simulink model "c00001M_harness"  (R2018a)
settings: Solver=ode3  StartTime=0.0  StopTime=10.0  RelTol=1e-3  EnableMultiTasking=on
undefined symbols (not defined in the file): b, DiscIntNeverNeededParam, J, K, L, R, sigbuilder_block
settings Model: Creator=aarrieta  LastModifiedBy=umarkiegi
settings DataIOCC: LimitDataPoints=on  SaveFormat=Array
settings OptimizationCC: LifeSpan=inf
settings DebuggingCC: UnderspecifiedInitializationDetection=Classic  MergeDetectMultiDrivingBlocksExec=none  SolverPrmCheckMsg=warning  StateNameClashWarn=warning  SFUnexpectedBacktrackingDiag=warning  SFNoUnconditionalDefaultTransitionDiag=warning  SFExecutionAtInitializationDiag=none
settings HardwareCC: ProdBitPerPointer=32  ProdBitPerSizeT=32  ProdBitPerPtrDiffT=32  ProdLargestAtomicFloat=None  ProdIntDivRoundTo=Undefined  ProdEndianess=Unspecified  ProdWordSize=32  ProdHWDeviceType=32-bit Generic
settings ModelReferenceCC: PropagateSignalLabelsOutOfModel=off
settings CodeAppCC: StateflowObjectComments=on
settings GRTTargetCC: TargetLangStandard=C89/C90 (ANSI)  GeneratePreprocessorConditionals=Disable all
settings ConfigComp: CovMetricSettings=dw  CovHtmlReporting=on  CovSaveCumulativeToWorkspaceVar=on  CovSaveSingleToWorkspaceVar=on  CovExternalEMLEnable=off  DVMaxTestCaseSteps=20  DVTestSuiteOptimization=CombinedObjectives (Nonlinear Extended)  DVDetectFloatOverflow=off

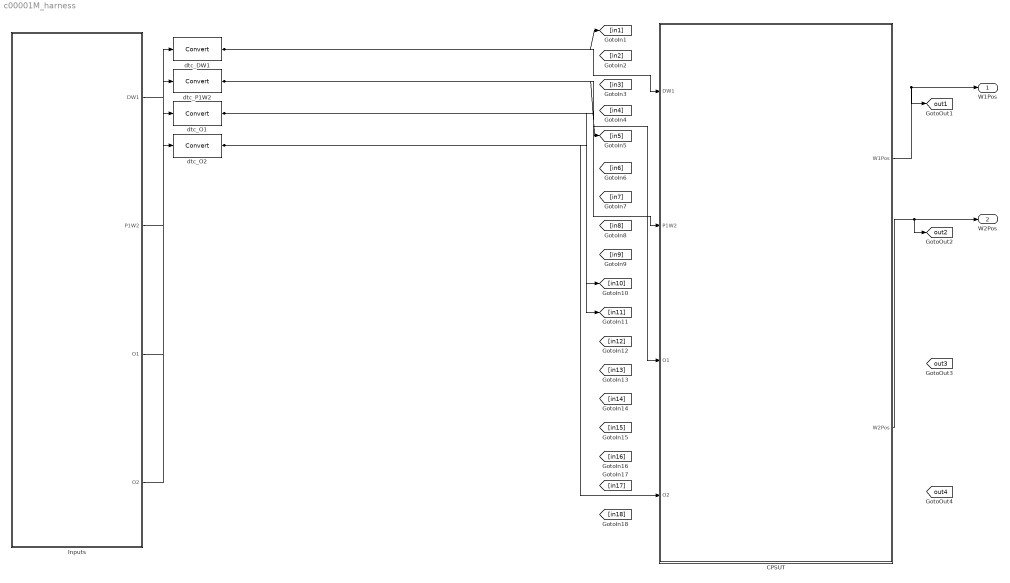
== system c00001M_harness ==
  CPSUT : Subsystem
  Inputs : Subsystem  Tag=STV Subsys  LoadFcn=sigbuilder_block('load');  StartFcn=sigbuilder_block('start');  StopFcn=sigbuilder_block('stop');  ClipboardFcn=sigbuilder_block('clipboard');  mask(Sigbuilder block){tuvar=[0:10]}
      mask init:
      | if ~strcmp(get_param(bdroot(gcb),'SimulationStatus'),'stopped'),tuvar = sigbuilder_block('maskInit'); end
      settings: CopyFcn=sigbuilder_block('copy');  DeleteFcn=sigbuilder_block('delete');  ModelCloseFcn=sigbuilder_block('modelClose');  PreSaveFcn=sigbuilder_block('preSave');  PauseFcn=sigbuilder_block('pause');  ContinueFcn=sigbuilder_block('continue');  NameChangeFcn=sigbuilder_block('namechange');  OpenFcn=sigbuilder_block('open');  CloseFcn=sigbuilder_block('close');
      mask Display: plot(0, 0, 100, 100,[2, 2, 32, 32, 2], [68, 8, 8, 68, 68],[32, 2], [38, 38], [32, 19, 2],[53, 60, 44], [32, 17, 17, 2],[16, 16, 31, 31]);txt = getActiveGroup(gcbh);text(2, 100, txt,'verticalAlignment', 'top');
  dtc_DW1 : DataTypeConversion
  dtc_O1 : DataTypeConversion
  dtc_O2 : DataTypeConversion
  dtc_P1W2 : DataTypeConversion
  W1Pos : Outport
  W2Pos : Outport  Port=2
  tag scope: out1=global, out2=global, out3=global, out4=global
  wires:
  CPSUT/2(W2Pos) -> [out2], W2Pos/1
  CPSUT/1(W1Pos) -> [out1], W1Pos/1
  Inputs/1(DW1) -> dtc_DW1/1
  dtc_DW1/1 -> CPSUT/1(DW1), [in1]
  Inputs/2(P1W2) -> dtc_P1W2/1
  dtc_P1W2/1 -> CPSUT/2(P1W2), [in5]
  Inputs/3(O1) -> dtc_O1/1
  dtc_O1/1 -> CPSUT/3(O1), [in10]
  Inputs/4(O2) -> dtc_O2/1
  dtc_O2/1 -> CPSUT/4(O2), [in11]

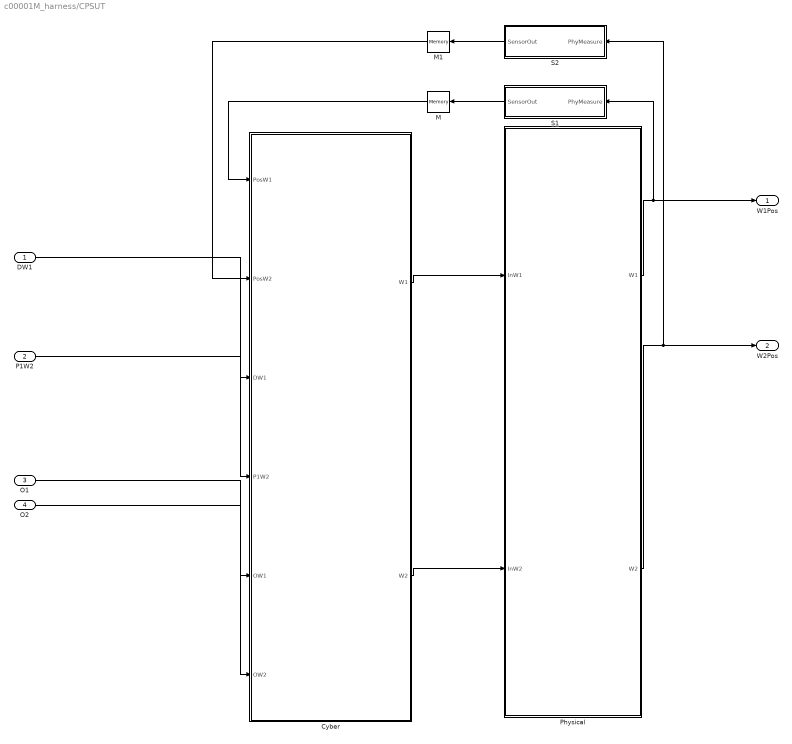
== system c00001M_harness/CPSUT ==
  DW1 : Inport  OutMin=0  OutMax=4  OutDataTypeStr=int8
  P1W2 : Inport  Port=2  OutMin=0  OutMax=4  OutDataTypeStr=int8
  O1 : Inport  Port=3  OutDataTypeStr=boolean
  O2 : Inport  Port=4  OutDataTypeStr=boolean
  Cyber : Subsystem
  M : Memory
  M1 : Memory
  Physical : Subsystem
  S1 : Subsystem
  S2 : Subsystem
  W1Pos : Outport
  W2Pos : Outport  Port=2
  wires:
  S1/1(SensorOut) -> M/1
  Physical/1(W1) -> W1Pos/1, S1/1(PhyMeasure)
  O2/1 -> Cyber/6(OW2)
  O1/1 -> Cyber/5(OW1)
  Cyber/1(W1) -> Physical/1(InW1)
  Cyber/2(W2) -> Physical/2(InW2)
  P1W2/1 -> Cyber/4(P1W2)
  M1/1 -> Cyber/2(PosW2)
  M/1 -> Cyber/1(PosW1)
  DW1/1 -> Cyber/3(DW1)
  Physical/2(W2) -> W2Pos/1, S2/1(PhyMeasure)
  S2/1(SensorOut) -> M1/1

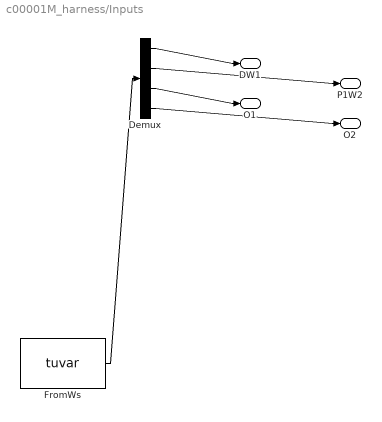
== system c00001M_harness/Inputs ==
  Demux : Demux  Tag=STV Demux
  FromWs : FromWorkspace  Tag=STV FromWs  VariableName=tuvar  SampleTime=0
      SigBuilderData=|
      | dataSet(1).timeRange = [0 20]
      | dataSet(1).name = 'Test Case 1'
      | dataSet(2).timeRange = [0 10]
      | dataSet(2).name = 'Test Case 2'
      | dataSet(3).timeRange = [0 8]
      | dataSet(3).name = 'Test Case 3'
      | dataSet(4).timeRange = [0 6]
      | dataSet(4).name = 'Test Case 4'
      | dataSet(5).timeRange = [0 6]
      | dataSet(5).name = 'Test Case 5'
      | dataSet(6).timeRange = [0 6]
      | dataSet(6).name = 'Test Case 6'
      | dataSet(7).timeRange = [0 8]
      | dataSet(7).name = 'Test Case 7'
      | dataSet(8).timeRange = [0 6]
      | dataSet(8).name = 'Test Case 8'
      | dataSet(9).timeRange = [0 6]
      | dataSet(9).name = 'Test Case 9'
      | dataSet(10).timeRange = [0 7]
      | dataSet(10).name = 'Test Case 10'
      | dataSet(11).timeRange = [0 9]
      | dataSet(11).name = 'Test Case 11'
      | dataSet(12).timeRange = [0 8]
      | dataSet(12).name = 'Test Case 12'
      | dataSet(13).timeRange = [0 12]
      | dataSet(13).name = 'Test Case 13'
      | dataSet(14).timeRange = [0 8]
      | dataSet(14).name = 'Test Case 14'
      | dataSet(15).timeRange = [0 8]
      | dataSet(15).name = 'Test Case 15'
      | dataSet(16).timeRange = [0 8]
      | dataSet(16).name = 'Test Case 16'
      | dataSet(17).timeRange = [0 8]
      | dataSet(17).name = 'Test Case 17'
      | dataSet(18).timeRange = [0 8]
      | dataSet(18).name = 'Test Case 18'
      | dataSet(19).timeRange = [0 8]
      | dataSet(19).name = 'Test Case 19'
      | dataSet(20).timeRange = [0 7]
      | dataSet(20).name = 'Test Case 20'
      | dataSet(21).timeRange = [0 7]
      | dataSet(21).name = 'Test Case 21'
      | dataSet(22).timeRange = [0 7]
      | dataSet(22).name = 'Test Case 22'
      | dataSet(23).timeRange = [0 8]
      | dataSet(23).name = 'Test Case 23'
      | dataSet(24).timeRange = [0 8]
      | dataSet(24).name = 'Test Case 24'
      | dataSet(25).timeRange = [0 8]
      | dataSet(25).name = 'Test Case 25'
      | dataSet(26).timeRange = [0 8]
      | dataSet(26).name = 'Test Case 26'
      | sbobj.Name = 'Signal Builder'
      | sbobj.Groups(1).Name = 'Test Case 1'
      | sbobj.Groups(1).Signals(1).Name = 'DW1'
      | sbobj.Groups(1).Signals(1).XData = [0 2 8 11 11 13 16 17 17 19 19 20]
      | sbobj.Groups(1).Signals(1).YData = [1 1 1 1 0 0 0 0 4 4 3 3]
      | sbobj.Groups(1).Signals(2).Name = 'P1W2'
      | sbobj.Groups(1).Signals(2).XData = [0 2 2 8 8 11 11 13 13 16 16 17 17 19 19 20]
      | sbobj.Groups(1).Signals(2).YData = [2 2 2 2 4 4 3 3 1 1 0 0 0 0 0 0]
      | sbobj.Groups(1).Signals(3).Name = 'O1'
      | sbobj.Groups(1).Signals(3).XData = [0 2 2 8 8 11 11 13 13 16 16 17 17 19 19 20]
      | sbobj.Groups(1).Signals(3).YData = [1 1 1 1 1 1 1 1 1 1 0 0 0 0 0 0]
      | sbobj.Groups(1).Signals(4).Name = 'O2'
      | sbobj.Groups(1).Signals(4).XData = [0 2 2 8 8 11 11 13 13 16 16 17 17 19 19 20]
      | sbobj.Groups(1).Signals(4).YData = [0 0 1 1 0 0 0 0 0 0 0 0 0 0 0 0]
      | sbobj.Groups(1).TimeRange = [0 20]
      | sbobj.Groups(2).Name = 'Test Case 2'
      | sbobj.Groups(2).Signals(1).Name = 'DW1'
      | sbobj.Groups(2).Signals(1).XData = [0 3 3 5 5 9 9 10]
      | sbobj.Groups(2).Signals(1).YData = [3 3 3 3 2 2 2 2]
      | sbobj.Groups(2).Signals(2).Name = 'P1W2'
      | sbobj.Groups(2).Signals(2).XData = [0 3 3 5 5 9 9 10]
      | sbobj.Groups(2).Signals(2).YData = [3 3 0 0 0 0 1 1]
      | sbobj.Groups(2).Signals(3).Name = 'O1'
      | sbobj.Groups(2).Signals(3).XData = [0 3 3 5 5 9 9 10]
      | sbobj.Groups(2).Signals(3).YData = [1 1 1 1 0 0 0 0]
      | sbobj.Groups(2).Signals(4).Name = 'O2'
      | sbobj.Groups(2).Signals(4).XData = [0 3 3 5 5 9 9 10]
      | sbobj.Groups(2).Signals(4).YData = [0 0 0 0 0 0 0 0]
      | sbobj.Groups(3).Name = 'Test Case 3'
      | sbobj.Groups(3).Signals(1).Name = 'DW1'
      | sbobj.Groups(3).Signals(1).XData = [0 3 3 4 4 7 7 8]
      | sbobj.Groups(3).Signals(1).YData = [4 4 0 0 1 1 1 1]
      | sbobj.Groups(3).Signals(2).Name = 'P1W2'
      | sbobj.Groups(3).Signals(2).XData = [0 3 3 4 4 7 7 8]
      | sbobj.Groups(3).Signals(2).YData = [4 4 1 1 0 0 3 3]
      | sbobj.Groups(3).Signals(3).Name = 'O1'
      | sbobj.Groups(3).Signals(3).XData = [0 3 3 4 4 7 7 8]
      | sbobj.Groups(3).Signals(3).YData = [0 0 0 0 0 0 0 0]
      | sbobj.Groups(3).Signals(4).Name = 'O2'
      | sbobj.Groups(3).Signals(4).XData = [0 3 3 4 4 7 7 8]
      | sbobj.Groups(3).Signals(4).YData = [0 0 0 0 0 0 0 0]
      | sbobj.Groups(3).TimeRange = [0 8]
      | sbobj.Groups(4).Name = 'Test Case 4'
      | sbobj.Groups(4).Signals(1).Name = 'DW1'
      | sbobj.Groups(4).Signals(1).XData = [0 3 3 5 5 6]
      | sbobj.Groups(4).Signals(1).YData = [4 4 2 2 2 2]
      | sbobj.Groups(4).Signals(2).Name = 'P1W2'
      | sbobj.Groups(4).Signals(2).XData = [0 3 3 5 5 6]
      | sbobj.Groups(4).Signals(2).YData = [1 1 0 0 0 0]
      | sbobj.Groups(4).Signals(3).Name = 'O1'
      | sbobj.Groups(4).Signals(3).XData = [0 3 3 5 5 6]
      | sbobj.Groups(4).Signals(3).YData = [0 0 0 0 0 0]
      | sbobj.Groups(4).Signals(4).Name = 'O2'
      | sbobj.Groups(4).Signals(4).XData = [0 3 3 5 5 6]
      | sbobj.Groups(4).Signals(4).YData = [0 0 0 0 1 1]
      | sbobj.Groups(4).TimeRange = [0 6]
      | sbobj.Groups(5).Name = 'Test Case 5'
      | sbobj.Groups(5).Signals(1).Name = 'DW1'
      | sbobj.Groups(5).Signals(1).XData = [0 3 3 5 5 6]
      | sbobj.Groups(5).Signals(1).YData = [3 3 0 0 3 3]
      | sbobj.Groups(5).Signals(2).Name = 'P1W2'
      | sbobj.Groups(5).Signals(2).XData = [0 3 3 5 5 6]
      | sbobj.Groups(5).Signals(2).YData = [4 4 0 0 3 3]
      | sbobj.Groups(5).Signals(3).Name = 'O1'
      | sbobj.Groups(5).Signals(3).XData = [0 3 3 5 5 6]
      | sbobj.Groups(5).Signals(3).YData = [0 0 0 0 1 1]
      | sbobj.Groups(5).Signals(4).Name = 'O2'
      | sbobj.Groups(5).Signals(4).XData = [0 3 3 5 5 6]
      | sbobj.Groups(5).Signals(4).YData = [1 1 0 0 0 0]
      | sbobj.Groups(5).TimeRange = [0 6]
      | sbobj.Groups(6).Name = 'Test Case 6'
      | sbobj.Groups(6).Signals(1).Name = 'DW1'
      | sbobj.Groups(6).Signals(1).XData = [0 3 3 5 5 6]
      | sbobj.Groups(6).Signals(1).YData = [1 1 1 1 0 0]
      | sbobj.Groups(6).Signals(2).Name = 'P1W2'
      | sbobj.Groups(6).Signals(2).XData = [0 3 3 5 5 6]
      | sbobj.Groups(6).Signals(2).YData = [4 4 2 2 0 0]
      | sbobj.Groups(6).Signals(3).Name = 'O1'
      | sbobj.Groups(6).Signals(3).XData = [0 3 3 5 5 6]
      | sbobj.Groups(6).Signals(3).YData = [1 1 1 1 1 1]
      | sbobj.Groups(6).Signals(4).Name = 'O2'
      | sbobj.Groups(6).Signals(4).XData = [0 3 3 5 5 6]
      | sbobj.Groups(6).Signals(4).YData = [0 0 0 0 1 1]
      | sbobj.Groups(6).TimeRange = [0 6]
      | sbobj.Groups(7).Name = 'Test Case 7'
      | sbobj.Groups(7).Signals(1).Name = 'DW1'
      | sbobj.Groups(7).Signals(1).XData = [0 3 3 4 4 7 7 8]
      | sbobj.Groups(7).Signals(1).YData = [1 1 1 1 1 1 3 3]
      | sbobj.Groups(7).Signals(2).Name = 'P1W2'
      | sbobj.Groups(7).Signals(2).XData = [0 3 3 4 4 7 7 8]
      | sbobj.Groups(7).Signals(2).YData = [4 4 3 3 2 2 0 0]
      | sbobj.Groups(7).Signals(3).Name = 'O1'
      | sbobj.Groups(7).Signals(3).XData = [0 3 3 4 4 7 7 8]
      | sbobj.Groups(7).Signals(3).YData = [1 1 1 1 1 1 0 0]
      | sbobj.Groups(7).Signals(4).Name = 'O2'
      | sbobj.Groups(7).Signals(4).XData = [0 3 3 4 4 7 7 8]
      | sbobj.Groups(7).Signals(4).YData = [0 0 0 0 0 0 1 1]
      | sbobj.Groups(7).TimeRange = [0 8]
      | sbobj.Groups(8).Name = 'Test Case 8'
      | sbobj.Groups(8).Signals(1).Name = 'DW1'
      | sbobj.Groups(8).Signals(1).XData = [0 2 2 3 3 5 5 6]
      | sbobj.Groups(8).Signals(1).YData = [1 1 2 2 2 2 2 2]
      | sbobj.Groups(8).Signals(2).Name = 'P1W2'
      | sbobj.Groups(8).Signals(2).XData = [0 2 2 3 3 5 5 6]
      | sbobj.Groups(8).Signals(2).YData = [4 4 3 3 1 1 3 3]
      | sbobj.Groups(8).Signals(3).Name = 'O1'
      | sbobj.Groups(8).Signals(3).XData = [0 2 2 3 3 5 5 6]
      | sbobj.Groups(8).Signals(3).YData = [1 1 1 1 1 1 0 0]
      | sbobj.Groups(8).Signals(4).Name = 'O2'
      | sbobj.Groups(8).Signals(4).XData = [0 2 2 3 3 5 5 6]
      | sbobj.Groups(8).Signals(4).YData = [0 0 1 1 0 0 0 0]
      | sbobj.Groups(8).TimeRange = [0 6]
      | sbobj.Groups(9).Name = 'Test Case 9'
      | sbobj.Groups(9).Signals(1).Name = 'DW1'
      | sbobj.Groups(9).Signals(1).XData = [0 2 2 3 3 5 5 6]
      | sbobj.Groups(9).Signals(1).YData = [1 1 4 4 3 3 2 2]
      | sbobj.Groups(9).Signals(2).Name = 'P1W2'
      | sbobj.Groups(9).Signals(2).XData = [0 2 2 3 3 5 5 6]
      | sbobj.Groups(9).Signals(2).YData = [4 4 0 0 0 0 1 1]
      | sbobj.Groups(9).Signals(3).Name = 'O1'
      | sbobj.Groups(9).Signals(3).XData = [0 2 2 3 3 5 5 6]
      | sbobj.Groups(9).Signals(3).YData = [1 1 1 1 0 0 1 1]
      | sbobj.Groups(9).Signals(4).Name = 'O2'
      | sbobj.Groups(9).Signals(4).XData = [0 2 2 3 3 5 5 6]
      | sbobj.Groups(9).Signals(4).YData = [0 0 1 1 0 0 1 1]
      | sbobj.Groups(9).TimeRange = [0 6]
      | sbobj.Groups(10).Name = 'Test Case 10'
      | sbobj.Groups(10).Signals(1).Name = 'DW1'
      | sbobj.Groups(10).Signals(1).XData = [0 2 2 3 3 6 6 7]
      | sbobj.Groups(10).Signals(1).YData = [1 1 3 3 2 2 0 0]
      | sbobj.Groups(10).Signals(2).Name = 'P1W2'
      | sbobj.Groups(10).Signals(2).XData = [0 2 2 3 3 6 6 7]
      | sbobj.Groups(10).Signals(2).YData = [4 4 0 0 0 0 1 1]
      | sbobj.Groups(10).Signals(3).Name = 'O1'
      | sbobj.Groups(10).Signals(3).XData = [0 2 2 3 3 6 6 7]
      | sbobj.Groups(10).Signals(3).YData = [1 1 1 1 0 0 0 0]
      | sbobj.Groups(10).Signals(4).Name = 'O2'
      | sbobj.Groups(10).Signals(4).XData = [0 2 2 3 3 6 6 7]
      | sbobj.Groups(10).Signals(4).YData = [0 0 1 1 0 0 0 0]
      | sbobj.Groups(10).TimeRange = [0 7]
      | sbobj.Groups(11).Name = 'Test Case 11'
      | sbobj.Groups(11).Signals(1).Name = 'DW1'
      | sbobj.Groups(11).Signals(1).XData = [0 4 4 5 5 7 7 8 8 9]
      | sbobj.Groups(11).Signals(1).YData = [3 3 1 1 0 0 2 2 3 3]
      | sbobj.Groups(11).Signals(2).Name = 'P1W2'
      | sbobj.Groups(11).Signals(2).XData = [0 4 4 5 5 7 7 8 8 9]
      | sbobj.Groups(11).Signals(2).YData = [4 4 0 0 0 0 2 2 3 3]
      | sbobj.Groups(11).Signals(3).Name = 'O1'
      | sbobj.Groups(11).Signals(3).XData = [0 4 4 5 5 7 7 8 8 9]
      | sbobj.Groups(11).Signals(3).YData = [0 0 0 0 0 0 0 0 1 1]
      | sbobj.Groups(11).Signals(4).Name = 'O2'
      | sbobj.Groups(11).Signals(4).XData = [0 4 4 5 5 7 7 8 8 9]
      | sbobj.Groups(11).Signals(4).YData = [1 1 0 0 0 0 0 0 1 1]
      | sbobj.Groups(11).TimeRange = [0 9]
      | sbobj.Groups(12).Name = 'Test Case 12'
      | sbobj.Groups(12).Signals(1).Name = 'DW1'
      | sbobj.Groups(12).Signals(1).XData = [0 4 4 6 6 7 7 8]
      | sbobj.Groups(12).Signals(1).YData = [3 3 4 4 1 1 3 3]
      | sbobj.Groups(12).Signals(2).Name = 'P1W2'
      | sbobj.Groups(12).Signals(2).XData = [0 4 4 6 6 7 7 8]
      | sbobj.Groups(12).Signals(2).YData = [4 4 0 0 1 1 2 2]
      | sbobj.Groups(12).Signals(3).Name = 'O1'
      | sbobj.Groups(12).Signals(3).XData = [0 4 4 6 6 7 7 8]
      | sbobj.Groups(12).Signals(3).YData = [0 0 0 0 1 1 0 0]
      | sbobj.Groups(12).Signals(4).Name = 'O2'
      | sbobj.Groups(12).Signals(4).XData = [0 4 4 6 6 7 7 8]
      | sbobj.Groups(12).Signals(4).YData = [1 1 0 0 0 0 1 1]
      | sbobj.Groups(12).TimeRange = [0 8]
      | sbobj.Groups(13).Name = 'Test Case 13'
      | sbobj.Groups(13).Signals(1).Name = 'DW1'
      | sbobj.Groups(13).Signals(1).XData = [0 2 2 3 3 5 5 6 6 8 8 11 11 12]
      | sbobj.Groups(13).Signals(1).YData = [4 4 4 4 0 0 1 1 1 1 4 4 2 2]
      | sbobj.Groups(13).Signals(2).Name = 'P1W2'
      | sbobj.Groups(13).Signals(2).XData = [0 2 2 3 3 5 5 6 6 8 8 11 11 12]
      | sbobj.Groups(13).Signals(2).YData = [1 1 3 3 4 4 2 2 3 3 0 0 1 1]
      | sbobj.Groups(13).Signals(3).Name = 'O1'
      | sbobj.Groups(13).Signals(3).XData = [0 2 2 3 3 5 5 6 6 8 8 11 11 12]
      | sbobj.Groups(13).Signals(3).YData = [0 0 1 1 1 1 1 1 1 1 1 1 0 0]
      | sbobj.Groups(13).Signals(4).Name = 'O2'
      | sbobj.Groups(13).Signals(4).XData = [0 2 2 3 3 5 5 6 6 8 8 11 11 12]
      | sbobj.Groups(13).Signals(4).YData = [0 0 1 1 0 0 0 0 0 0 0 0 1 1]
      | sbobj.Groups(13).TimeRange = [0 12]
      | sbobj.Groups(14).Name = 'Test Case 14'
      | sbobj.Groups(14).Signals(1).Name = 'DW1'
      | sbobj.Groups(14).Signals(1).XData = [0 3 3 4 4 5 5 7 7 8]
      | sbobj.Groups(14).Signals(1).YData = [4 4 0 0 1 1 4 4 3 3]
      | sbobj.Groups(14).Signals(2).Name = 'P1W2'
      | sbobj.Groups(14).Signals(2).XData = [0 3 3 4 4 5 5 7 7 8]
      | sbobj.Groups(14).Signals(2).YData = [4 4 1 1 0 0 0 0 2 2]
      | sbobj.Groups(14).Signals(3).Name = 'O1'
      | sbobj.Groups(14).Signals(3).XData = [0 3 3 4 4 5 5 7 7 8]
      | sbobj.Groups(14).Signals(3).YData = [0 0 0 0 0 0 0 0 0 0]
      | sbobj.Groups(14).Signals(4).Name = 'O2'
      | sbobj.Groups(14).Signals(4).XData = [0 3 3 4 4 5 5 7 7 8]
      | sbobj.Groups(14).Signals(4).YData = [0 0 0 0 0 0 0 0 1 1]
      | sbobj.Groups(14).TimeRange = [0 8]
      | sbobj.Groups(15).Name = 'Test Case 15'
      | sbobj.Groups(15).Signals(1).Name = 'DW1'
      | sbobj.Groups(15).Signals(1).XData = [0 3 3 4 4 5 5 7 7 8]
      | sbobj.Groups(15).Signals(1).YData = [4 4 0 0 1 1 3 3 0 0]
      | sbobj.Groups(15).Signals(2).Name = 'P1W2'
      | sbobj.Groups(15).Signals(2).XData = [0 3 3 4 4 5 5 7 7 8]
      | sbobj.Groups(15).Signals(2).YData = [4 4 1 1 0 0 0 0 0 0]
      | sbobj.Groups(15).Signals(3).Name = 'O1'
      | sbobj.Groups(15).Signals(3).XData = [0 3 3 4 4 5 5 7 7 8]
      | sbobj.Groups(15).Signals(3).YData = [0 0 0 0 0 0 0 0 1 1]
      | sbobj.Groups(15).Signals(4).Name = 'O2'
      | sbobj.Groups(15).Signals(4).XData = [0 3 3 4 4 5 5 7 7 8]
      | sbobj.Groups(15).Signals(4).YData = [0 0 0 0 0 0 0 0 1 1]
      | sbobj.Groups(15).TimeRange = [0 8]
      | sbobj.Groups(16).Name = 'Test Case 16'
      | sbobj.Groups(16).Signals(1).Name = 'DW1'
      | sbobj.Groups(16).Signals(1).XData = [0 3 3 4 4 5 5 7 7 8]
      | sbobj.Groups(16).Signals(1).YData = [4 4 0 0 1 1 2 2 3 3]
      | sbobj.Groups(16).Signals(2).Name = 'P1W2'
      | sbobj.Groups(16).Signals(2).XData = [0 3 3 4 4 5 5 7 7 8]
      | sbobj.Groups(16).Signals(2).YData = [4 4 1 1 0 0 0 0 4 4]
      | sbobj.Groups(16).Signals(3).Name = 'O1'
      | sbobj.Groups(16).Signals(3).XData = [0 3 3 4 4 5 5 7 7 8]
      | sbobj.Groups(16).Signals(3).YData = [0 0 0 0 0 0 0 0 0 0]
      | sbobj.Groups(16).Signals(4).Name = 'O2'
      | sbobj.Groups(16).Signals(4).XData = [0 3 3 4 4 5 5 7 7 8]
      | sbobj.Groups(16).Signals(4).YData = [0 0 0 0 0 0 0 0 1 1]
      | sbobj.Groups(16).TimeRange = [0 8]
      | sbobj.Groups(17).Name = 'Test Case 17'
      | sbobj.Groups(17).Signals(1).Name = 'DW1'
      | sbobj.Groups(17).Signals(1).XData = [0 4 4 5 5 7 7 8]
      | sbobj.Groups(17).Signals(1).YData = [3 3 4 4 4 4 0 0]
      | sbobj.Groups(17).Signals(2).Name = 'P1W2'
      | sbobj.Groups(17).Signals(2).XData = [0 4 4 5 5 7 7 8]
      | sbobj.Groups(17).Signals(2).YData = [3 3 2 2 4 4 3 3]
      | sbobj.Groups(17).Signals(3).Name = 'O1'
      | sbobj.Groups(17).Signals(3).XData = [0 4 4 5 5 7 7 8]
      | sbobj.Groups(17).Signals(3).YData = [1 1 1 1 1 1 0 0]
      | sbobj.Groups(17).Signals(4).Name = 'O2'
      | sbobj.Groups(17).Signals(4).XData = [0 4 4 5 5 7 7 8]
      | sbobj.Groups(17).Signals(4).YData = [0 0 0 0 0 0 1 1]
      | sbobj.Groups(17).TimeRange = [0 8]
      | sbobj.Groups(18).Name = 'Test Case 18'
      | sbobj.Groups(18).Signals(1).Name = 'DW1'
      | sbobj.Groups(18).Signals(1).XData = [0 4 4 5 5 7 7 8]
      | sbobj.Groups(18).Signals(1).YData = [3 3 4 4 4 4 0 0]
      | sbobj.Groups(18).Signals(2).Name = 'P1W2'
      | sbobj.Groups(18).Signals(2).XData = [0 4 4 5 5 7 7 8]
      | sbobj.Groups(18).Signals(2).YData = [3 3 2 2 1 1 4 4]
      | sbobj.Groups(18).Signals(3).Name = 'O1'
      | sbobj.Groups(18).Signals(3).XData = [0 4 4 5 5 7 7 8]
      | sbobj.Groups(18).Signals(3).YData = [1 1 1 1 1 1 1 1]
      | sbobj.Groups(18).Signals(4).Name = 'O2'
      | sbobj.Groups(18).Signals(4).XData = [0 4 4 5 5 7 7 8]
      | sbobj.Groups(18).Signals(4).YData = [0 0 0 0 0 0 0 0]
      | sbobj.Groups(18).TimeRange = [0 8]
      | sbobj.Groups(19).Name = 'Test Case 19'
      | sbobj.Groups(19).Signals(1).Name = 'DW1'
      | sbobj.Groups(19).Signals(1).XData = [0 4 4 7 7 8]
      | sbobj.Groups(19).Signals(1).YData = [3 3 4 4 2 2]
      | sbobj.Groups(19).Signals(2).Name = 'P1W2'
      | sbobj.Groups(19).Signals(2).XData = [0 4 4 7 7 8]
      | sbobj.Groups(19).Signals(2).YData = [3 3 1 1 2 2]
      | sbobj.Groups(19).Signals(3).Name = 'O1'
      | sbobj.Groups(19).Signals(3).XData = [0 4 4 7 7 8]
      | sbobj.Groups(19).Signals(3).YData = [1 1 0 0 1 1]
      | sbobj.Groups(19).Signals(4).Name = 'O2'
      | sbobj.Groups(19).Signals(4).XData = [0 4 4 7 7 8]
      | sbobj.Groups(19).Signals(4).YData = [0 0 0 0 1 1]
      | sbobj.Groups(19).TimeRange = [0 8]
      | sbobj.Groups(20).Name = 'Test Case 20'
      | sbobj.Groups(20).Signals(1).Name = 'DW1'
      | sbobj.Groups(20).Signals(1).XData = [0 2 2 3 3 4 4 6 6 7]
      | sbobj.Groups(20).Signals(1).YData = [1 1 3 3 2 2 3 3 4 4]
      | sbobj.Groups(20).Signals(2).Name = 'P1W2'
      | sbobj.Groups(20).Signals(2).XData = [0 2 2 3 3 4 4 6 6 7]
      | sbobj.Groups(20).Signals(2).YData = [4 4 0 0 0 0 0 0 0 0]
      | sbobj.Groups(20).Signals(3).Name = 'O1'
      | sbobj.Groups(20).Signals(3).XData = [0 2 2 3 3 4 4 6 6 7]
      | sbobj.Groups(20).Signals(3).YData = [1 1 1 1 0 0 0 0 0 0]
      | sbobj.Groups(20).Signals(4).Name = 'O2'
      | sbobj.Groups(20).Signals(4).XData = [0 2 2 3 3 4 4 6 6 7]
      | sbobj.Groups(20).Signals(4).YData = [0 0 1 1 0 0 0 0 0 0]
      | sbobj.Groups(20).TimeRange = [0 7]
      | sbobj.Groups(21).Name = 'Test Case 21'
      | sbobj.Groups(21).Signals(1).Name = 'DW1'
      | sbobj.Groups(21).Signals(1).XData = [0 2 2 3 3 4 4 6 6 7]
      | sbobj.Groups(21).Signals(1).YData = [1 1 3 3 2 2 4 4 1 1]
      | sbobj.Groups(21).Signals(2).Name = 'P1W2'
      | sbobj.Groups(21).Signals(2).XData = [0 2 2 3 3 4 4 6 6 7]
      | sbobj.Groups(21).Signals(2).YData = [4 4 0 0 0 0 0 0 2 2]
      | sbobj.Groups(21).Signals(3).Name = 'O1'
      | sbobj.Groups(21).Signals(3).XData = [0 2 2 3 3 4 4 6 6 7]
      | sbobj.Groups(21).Signals(3).YData = [1 1 1 1 0 0 0 0 0 0]
      | sbobj.Groups(21).Signals(4).Name = 'O2'
      | sbobj.Groups(21).Signals(4).XData = [0 2 2 3 3 4 4 6 6 7]
      | sbobj.Groups(21).Signals(4).YData = [0 0 1 1 0 0 0 0 0 0]
      | sbobj.Groups(21).TimeRange = [0 7]
      | sbobj.Groups(22).Name = 'Test Case 22'
      | sbobj.Groups(22).Signals(1).Name = 'DW1'
      | sbobj.Groups(22).Signals(1).XData = [0 2 2 3 3 4 4 6 6 7]
      | sbobj.Groups(22).Signals(1).YData = [1 1 3 3 2 2 1 1 4 4]
      | sbobj.Groups(22).Signals(2).Name = 'P1W2'
      | sbobj.Groups(22).Signals(2).XData = [0 2 2 3 3 4 4 6 6 7]
      | sbobj.Groups(22).Signals(2).YData = [4 4 0 0 0 0 0 0 4 4]
      | sbobj.Groups(22).Signals(3).Name = 'O1'
      | sbobj.Groups(22).Signals(3).XData = [0 2 2 3 3 4 4 6 6 7]
      | sbobj.Groups(22).Signals(3).YData = [1 1 1 1 0 0 0 0 0 0]
      | sbobj.Groups(22).Signals(4).Name = 'O2'
      | sbobj.Groups(22).Signals(4).XData = [0 2 2 3 3 4 4 6 6 7]
      | sbobj.Groups(22).Signals(4).YData = [0 0 1 1 0 0 0 0 0 0]
      | sbobj.Groups(22).TimeRange = [0 7]
      | sbobj.Groups(23).Name = 'Test Case 23'
      | sbobj.Groups(23).Signals(1).Name = 'DW1'
      | sbobj.Groups(23).Signals(1).XData = [0 2 2 4 4 5 5 7 7 8]
      | sbobj.Groups(23).Signals(1).YData = [1 1 2 2 0 0 0 0 1 1]
      | sbobj.Groups(23).Signals(2).Name = 'P1W2'
      | sbobj.Groups(23).Signals(2).XData = [0 2 2 4 4 5 5 7 7 8]
      | sbobj.Groups(23).Signals(2).YData = [4 4 3 3 1 1 0 0 2 2]
      | sbobj.Groups(23).Signals(3).Name = 'O1'
      | sbobj.Groups(23).Signals(3).XData = [0 2 2 4 4 5 5 7 7 8]
      | sbobj.Groups(23).Signals(3).YData = [1 1 1 1 1 1 1 1 0 0]
      | sbobj.Groups(23).Signals(4).Name = 'O2'
      | sbobj.Groups(23).Signals(4).XData = [0 2 2 4 4 5 5 7 7 8]
      | sbobj.Groups(23).Signals(4).YData = [0 0 1 1 1 1 0 0 1 1]
      | sbobj.Groups(23).TimeRange = [0 8]
      | sbobj.Groups(24).Name = 'Test Case 24'
      | sbobj.Groups(24).Signals(1).Name = 'DW1'
      | sbobj.Groups(24).Signals(1).XData = [0 2 2 4 4 5 5 7 7 8]
      | sbobj.Groups(24).Signals(1).YData = [1 1 2 2 3 3 3 3 1 1]
      | sbobj.Groups(24).Signals(2).Name = 'P1W2'
      | sbobj.Groups(24).Signals(2).XData = [0 2 2 4 4 5 5 7 7 8]
      | sbobj.Groups(24).Signals(2).YData = [4 4 3 3 1 1 4 4 1 1]
      | sbobj.Groups(24).Signals(3).Name = 'O1'
      | sbobj.Groups(24).Signals(3).XData = [0 2 2 4 4 5 5 7 7 8]
      | sbobj.Groups(24).Signals(3).YData = [1 1 1 1 1 1 1 1 1 1]
      | sbobj.Groups(24).Signals(4).Name = 'O2'
      | sbobj.Groups(24).Signals(4).XData = [0 2 2 4 4 5 5 7 7 8]
      | sbobj.Groups(24).Signals(4).YData = [0 0 1 1 0 0 0 0 0 0]
      | sbobj.Groups(24).TimeRange = [0 8]
      | sbobj.Groups(25).Name = 'Test Case 25'
      | sbobj.Groups(25).Signals(1).Name = 'DW1'
      | sbobj.Groups(25).Signals(1).XData = [0 4 4 5 5 7 7 8]
      | sbobj.Groups(25).Signals(1).YData = [1 1 3 3 3 3 4 4]
      | sbobj.Groups(25).Signals(2).Name = 'P1W2'
      | sbobj.Groups(25).Signals(2).XData = [0 4 4 5 5 7 7 8]
      | sbobj.Groups(25).Signals(2).YData = [4 4 1 1 3 3 4 4]
      | sbobj.Groups(25).Signals(3).Name = 'O1'
      | sbobj.Groups(25).Signals(3).XData = [0 4 4 5 5 7 7 8]
      | sbobj.Groups(25).Signals(3).YData = [1 1 1 1 1 1 1 1]
      | sbobj.Groups(25).Signals(4).Name = 'O2'
      | sbobj.Groups(25).Signals(4).XData = [0 4 4 5 5 7 7 8]
      | sbobj.Groups(25).Signals(4).YData = [0 0 1 1 0 0 1 1]
      | sbobj.Groups(25).TimeRange = [0 8]
      | sbobj.Groups(26).Name = 'Test Case 26'
      | sbobj.Groups(26).Signals(1).Name = 'DW1'
      | sbobj.Groups(26).Signals(1).XData = [0 4 4 5 5 7 7 8]
      | sbobj.Groups(26).Signals(1).YData = [1 1 3 3 3 3 0 0]
      | sbobj.Groups(26).Signals(2).Name = 'P1W2'
      | sbobj.Groups(26).Signals(2).XData = [0 4 4 5 5 7 7 8]
      | sbobj.Groups(26).Signals(2).YData = [4 4 1 1 2 2 0 0]
      | sbobj.Groups(26).Signals(3).Name = 'O1'
      | sbobj.Groups(26).Signals(3).XData = [0 4 4 5 5 7 7 8]
      | sbobj.Groups(26).Signals(3).YData = [1 1 1 1 1 1 0 0]
      | sbobj.Groups(26).Signals(4).Name = 'O2'
      | sbobj.Groups(26).Signals(4).XData = [0 4 4 5 5 7 7 8]
      | sbobj.Groups(26).Signals(4).YData = [0 0 1 1 0 0 0 0]
      | sbobj.Groups(26).TimeRange = [0 8]
  DW1 : Outport  Tag=STV Outport
  P1W2 : Outport  Tag=STV Outport  Port=2
  O1 : Outport  Tag=STV Outport  Port=3
  O2 : Outport  Tag=STV Outport  Port=4
  wires:
  Demux/4 -> O2/1
  Demux/3 -> O1/1
  Demux/2 -> P1W2/1
  Demux/1 -> DW1/1
  FromWs/1 -> Demux/1

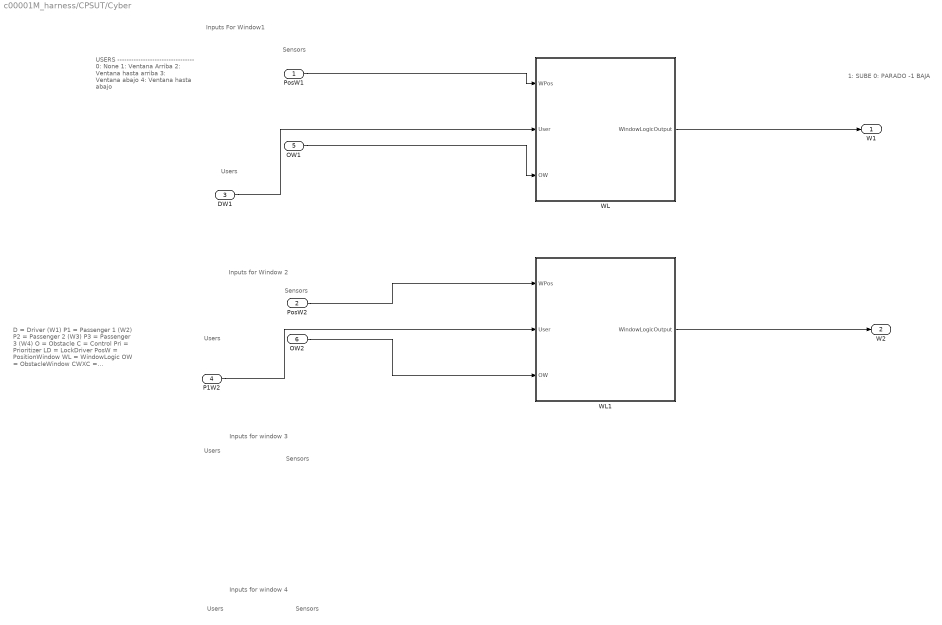
== system c00001M_harness/CPSUT/Cyber ==
  note: D = Driver (W1)
      | P1 = Passenger 1 (W2)
      | P2 = Passenger 2 (W3)
      | P3 = Passenger 3 (W4)
      | O = Obstacle
      | C = Control
      | Pri = Prioritizer
      | LD = LockDriver
      | PosW = PositionWindow
      | WL = WindowLogic
      | OW = ObstacleWindow
      | CWXC = ControlWindowXCentralized
      | S = Sensor
      | L = Lock
      | WPos = WindowPosition
      | M = Memory
      | InW = InputWindow
      | WIn = WindowInput
  note: 1: SUBE
      | 0: PARADO
      | -1 BAJA
  note: USERS
      | ---------------------------------
      | 0: None
      | 1: Ventana Arriba
      | 2: Ventana hasta arriba
      | 3: Ventana abajo
      | 4: Ventana hasta abajo
  note: Sensors
  note: Users
  note: Sensors
  note: Users
  note: Sensors
  note: Users
  note: Users
  note: Inputs for window 4
  note: Inputs for window 3
  note: Inputs for Window 2
  note: Inputs For Window1
  note: Sensors
  PosW1 : Inport
  PosW2 : Inport  Port=2
  DW1 : Inport  Port=3
  P1W2 : Inport  Port=4
  OW1 : Inport  Port=5
  OW2 : Inport  Port=6
  WL : Subsystem
  WL1 : Subsystem
  W1 : Outport
  W2 : Outport  Port=2
  wires:
  PosW1/1 -> WL/1(WPos)
  OW1/1 -> WL/3(OW)
  WL/1(WindowLogicOutput) -> W1/1
  PosW2/1 -> WL1/1(WPos)
  OW2/1 -> WL1/3(OW)
  WL1/1(WindowLogicOutput) -> W2/1
  DW1/1 -> WL/2(User)
  P1W2/1 -> WL1/2(User)

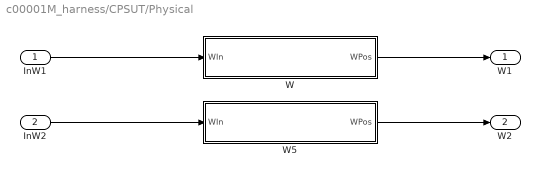
== system c00001M_harness/CPSUT/Physical ==
  InW1 : Inport
  InW2 : Inport  Port=2
  W : Subsystem
  W5 : Subsystem
  W1 : Outport
  W2 : Outport  Port=2
  wires:
  InW1/1 -> W/1(WIn)
  InW2/1 -> W5/1(WIn)
  W/1(WPos) -> W1/1
  W5/1(WPos) -> W2/1

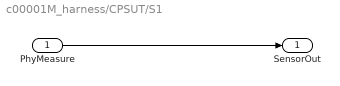
== system c00001M_harness/CPSUT/S1 ==
  PhyMeasure : Inport
  SensorOut : Outport
  wires:
  PhyMeasure/1 -> SensorOut/1

== system c00001M_harness/CPSUT/S2 ==
  PhyMeasure : Inport
  SensorOut : Outport
  wires:
  PhyMeasure/1 -> SensorOut/1

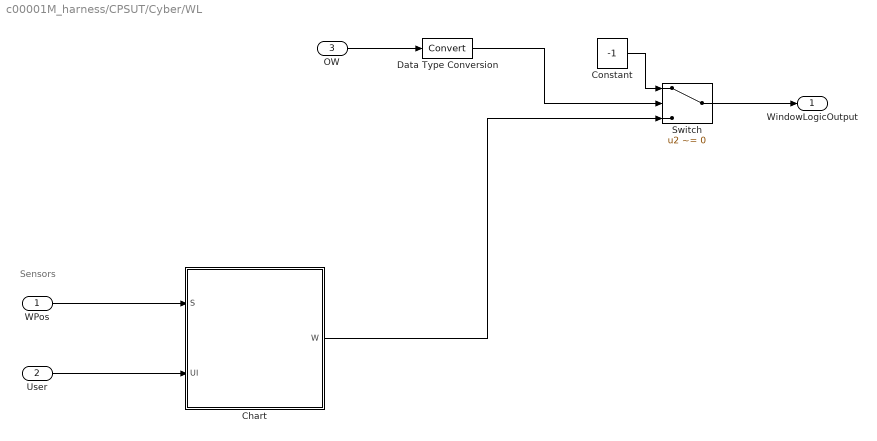
== system c00001M_harness/CPSUT/Cyber/WL ==
  note: Sensors
  WPos : Inport
  User : Inport  Port=2
  OW : Inport  Port=3
  Chart : Stateflow chart  TreatAsAtomicUnit=on
  Constant : Constant  Value=-1
  Data Type Conversion : DataTypeConversion
  Switch : Switch  Criteria=u2 ~= 0  Threshold=1  ZeroCross=off
  WindowLogicOutput : Outport
  wires:
  OW/1 -> Data Type Conversion/1
  Switch/1 -> WindowLogicOutput/1
  WPos/1 -> Chart/1(S)
  User/1 -> Chart/2(UI)
  Constant/1 -> Switch/1
  Data Type Conversion/1 -> Switch/2
  Chart/1(W) -> Switch/3

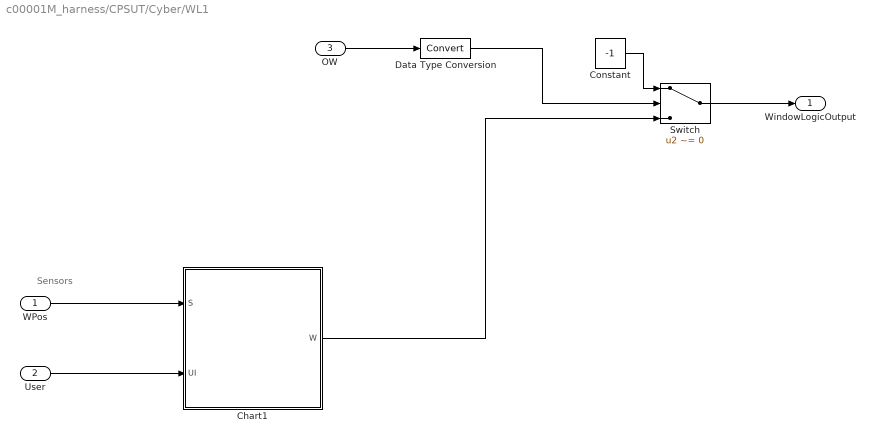
== system c00001M_harness/CPSUT/Cyber/WL1 ==
  note: Sensors
  WPos : Inport
  User : Inport  Port=2
  OW : Inport  Port=3
  Chart1 : Stateflow chart  TreatAsAtomicUnit=on
  Constant : Constant  Value=-1
  Data Type Conversion : DataTypeConversion
  Switch : Switch  Criteria=u2 ~= 0  Threshold=1  ZeroCross=off
  WindowLogicOutput : Outport
  wires:
  Data Type Conversion/1 -> Switch/2
  Constant/1 -> Switch/1
  User/1 -> Chart1/2(UI)
  WPos/1 -> Chart1/1(S)
  Switch/1 -> WindowLogicOutput/1
  OW/1 -> Data Type Conversion/1
  Chart1/1(W) -> Switch/3

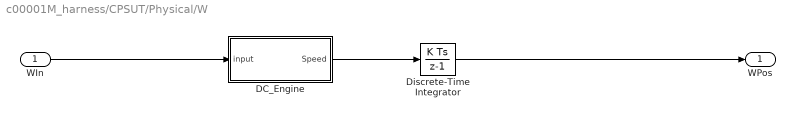
== system c00001M_harness/CPSUT/Physical/W ==
  WIn : Inport
  DC_Engine : Subsystem
  Discrete-Time Integrator : DiscreteIntegrator  InitialCondition=5  SampleTime=-1  LimitOutput=on  UpperSaturationLimit=5  LowerSaturationLimit=0  ICPrevOutput=DiscIntNeverNeededParam  ICPrevScaledInput=DiscIntNeverNeededParam
  WPos : Outport
  wires:
  Discrete-Time Integrator/1 -> WPos/1
  DC_Engine/1(Speed) -> Discrete-Time Integrator/1
  WIn/1 -> DC_Engine/1(input)

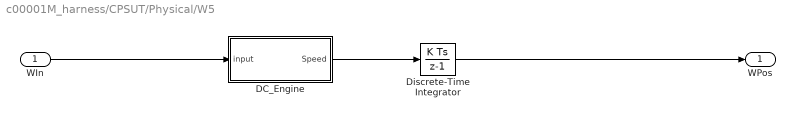
== system c00001M_harness/CPSUT/Physical/W5 ==
  WIn : Inport
  DC_Engine : Subsystem
  Discrete-Time Integrator : DiscreteIntegrator  InitialCondition=5  SampleTime=-1  LimitOutput=on  UpperSaturationLimit=5  LowerSaturationLimit=0  ICPrevOutput=DiscIntNeverNeededParam  ICPrevScaledInput=DiscIntNeverNeededParam
  WPos : Outport
  wires:
  WIn/1 -> DC_Engine/1(input)
  DC_Engine/1(Speed) -> Discrete-Time Integrator/1
  Discrete-Time Integrator/1 -> WPos/1

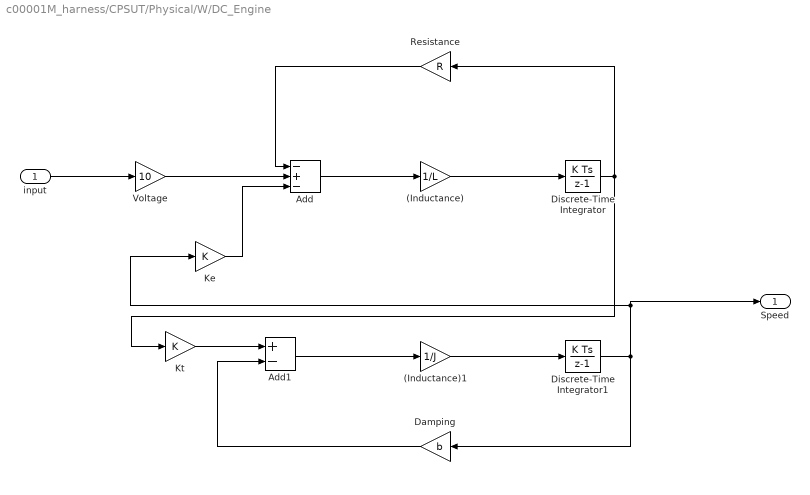
== system c00001M_harness/CPSUT/Physical/W/DC_Engine ==
  input : Inport
  (Inductance) : Gain  Gain=1/L
  (Inductance)1 : Gain  Gain=1/J
  Add : Sum  Inputs=-+-
  Add1 : Sum  Inputs=+-
  Damping : Gain  Gain=b
  Discrete-Time Integrator : DiscreteIntegrator  SampleTime=-1  ICPrevOutput=DiscIntNeverNeededParam  ICPrevScaledInput=DiscIntNeverNeededParam
  Discrete-Time Integrator1 : DiscreteIntegrator  SampleTime=-1  ICPrevOutput=DiscIntNeverNeededParam  ICPrevScaledInput=DiscIntNeverNeededParam
  Ke : Gain  Gain=K
  Kt : Gain  Gain=K
  Resistance : Gain  Gain=R
  Voltage : Gain  Gain=10
  Speed : Outport
  wires:
  input/1 -> Voltage/1
  Voltage/1 -> Add/2
  Add/1 -> (Inductance)/1
  Discrete-Time Integrator/1 -> Kt/1, Resistance/1
  Resistance/1 -> Add/1
  Ke/1 -> Add/3
  Kt/1 -> Add1/1
  Add1/1 -> (Inductance)1/1
  (Inductance)1/1 -> Discrete-Time Integrator1/1
  Discrete-Time Integrator1/1 -> Ke/1, Speed/1, Damping/1
  Damping/1 -> Add1/2
  (Inductance)/1 -> Discrete-Time Integrator/1

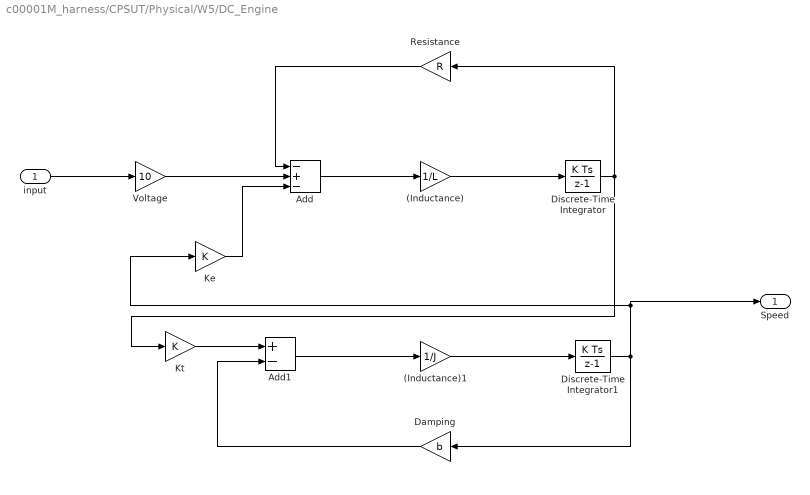
== system c00001M_harness/CPSUT/Physical/W5/DC_Engine ==
  input : Inport
  (Inductance) : Gain  Gain=1/L
  (Inductance)1 : Gain  Gain=1/J
  Add : Sum  Inputs=-+-
  Add1 : Sum  Inputs=+-
  Damping : Gain  Gain=b
  Discrete-Time Integrator : DiscreteIntegrator  SampleTime=-1  ICPrevOutput=DiscIntNeverNeededParam  ICPrevScaledInput=DiscIntNeverNeededParam
  Discrete-Time Integrator1 : DiscreteIntegrator  SampleTime=-1  ICPrevOutput=DiscIntNeverNeededParam  ICPrevScaledInput=DiscIntNeverNeededParam
  Ke : Gain  Gain=K
  Kt : Gain  Gain=K
  Resistance : Gain  Gain=R
  Voltage : Gain  Gain=10
  Speed : Outport
  wires:
  Damping/1 -> Add1/2
  Discrete-Time Integrator1/1 -> Damping/1, Speed/1, Ke/1
  (Inductance)1/1 -> Discrete-Time Integrator1/1
  Add1/1 -> (Inductance)1/1
  Kt/1 -> Add1/1
  Ke/1 -> Add/3
  Resistance/1 -> Add/1
  Discrete-Time Integrator/1 -> Resistance/1, Kt/1
  (Inductance)/1 -> Discrete-Time Integrator/1
  Add/1 -> (Inductance)/1
  Voltage/1 -> Add/2
  input/1 -> Voltage/1

== stateflow chart c00001M_harness/CPSUT/Cyber/WL/Chart ==
  state Bajand_hasta_abajo
    entry: W = -1;
  state Bajando
    entry: W = -1;
  state Idle
    entry:W = 0;
  state Subiendo_hasta_arriba
    entry: W = 1;
  state Subiendo
    entry: W = 1;
  Subiendo -> Bajand_hasta_abajo [order 4] : [UI==4]
  Bajand_hasta_abajo -> Bajando [order 2] : [UI==3]
  Subiendo -> Bajando [order 3] : [UI==3]
  Bajando -> Bajand_hasta_abajo [order 2] : [UI==4]
  Idle -> Bajando [order 3] : [UI==3&&S>0]
  Subiendo_hasta_arriba -> Bajand_hasta_abajo [order 3] : [UI==4]
  Idle -> Bajand_hasta_abajo [order 4] : [UI==4&&S>0]
  Bajando -> Subiendo [order 3] : [UI==1]
  Subiendo_hasta_arriba -> Bajando [order 4] : [UI==3]
  Bajand_hasta_abajo -> Subiendo [order 4] : [UI==1]
  Bajand_hasta_abajo -> Idle [order 1] : [S<=0]
  Bajand_hasta_abajo -> Subiendo_hasta_arriba [order 3] : [UI==2]
  Bajando -> Idle [order 1] : [S<=0||UI==0]
  Bajando -> Subiendo_hasta_arriba [order 4] : [UI==2]
  (default) -> Idle
  Idle -> Subiendo_hasta_arriba [order 2] : [UI==2&&S<5]
  Idle -> Subiendo [order 1] : [UI == 1&&S<5]
  Subiendo -> Idle [order 1] : [S>=5||UI==0]
  Subiendo_hasta_arriba -> Idle [order 1] : [S >=5]
  Subiendo_hasta_arriba -> Subiendo [order 2] : [UI ==1]
  Subiendo -> Subiendo_hasta_arriba [order 2] : [UI==2]
  data: S input; UI input; W output double

== stateflow chart c00001M_harness/CPSUT/Cyber/WL1/Chart1 ==
  state Bajand_hasta_abajo
    entry: W = -1;
  state Bajando
    entry: W = -1;
  state Idle
    entry:W = 0;
  state Subiendo_hasta_arriba
    entry: W = 1;
  state Subiendo
    entry: W = 1;
  Subiendo -> Bajand_hasta_abajo [order 4] : [UI==4]
  Bajand_hasta_abajo -> Bajando [order 2] : [UI==3]
  Subiendo -> Bajando [order 3] : [UI==3]
  Bajando -> Bajand_hasta_abajo [order 2] : [UI==4]
  Idle -> Bajando [order 3] : [UI==3&&S>0]
  Subiendo_hasta_arriba -> Bajand_hasta_abajo [order 3] : [UI==4]
  Idle -> Bajand_hasta_abajo [order 4] : [UI==4&&S>0]
  Bajando -> Subiendo [order 3] : [UI==1]
  Subiendo_hasta_arriba -> Bajando [order 4] : [UI==3]
  Bajand_hasta_abajo -> Subiendo [order 4] : [UI==1]
  Bajand_hasta_abajo -> Idle [order 1] : [S<=0]
  Bajand_hasta_abajo -> Subiendo_hasta_arriba [order 3] : [UI==2]
  Bajando -> Idle [order 1] : [S<=0||UI==0]
  Bajando -> Subiendo_hasta_arriba [order 4] : [UI==2]
  (default) -> Idle
  Idle -> Subiendo_hasta_arriba [order 2] : [UI==2&&S<5]
  Idle -> Subiendo [order 1] : [UI == 1&&S<5]
  Subiendo -> Idle [order 1] : [S>=5||UI==0]
  Subiendo_hasta_arriba -> Idle [order 1] : [S >=5]
  Subiendo_hasta_arriba -> Subiendo [order 2] : [UI ==1]
  Subiendo -> Subiendo_hasta_arriba [order 2] : [UI==2]
  data: S input; UI input; W output double
